simulink model "UnstablePlant"  (R2017b)
settings: Solver=VariableStepAuto  StartTime=0.0  StopTime=10.0  RelTol=1e-3
values from neighbouring files (symbols this model uses):
  Kp = 0.3    [open_loop.m]
  Ts = 0.005    [closed_loop.m]    (also in open_loop.m)
settings Model: Creator=tomas  LastModifiedBy=tomas

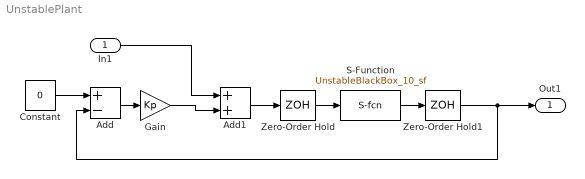
== system UnstablePlant ==
  In1 : Inport
  Add : Sum  Inputs=+-
  Add1 : Sum
  Constant : Constant  Value=0
  Gain : Gain  Gain=Kp
  S-Function : S-Function  FunctionName=UnstableBlackBox_10_sf  SFunctionDeploymentMode=off  EnableBusSupport=off  SFcnStateName=DWORK0
      settings: SFcnIsStateOwnerBlock=on
  Zero-Order Hold : ZeroOrderHold  SampleTime=Ts
  Zero-Order Hold1 : ZeroOrderHold  SampleTime=Ts
  Out1 : Outport
  wires:
  S-Function/1 -> Zero-Order Hold1/1
  Zero-Order Hold/1 -> S-Function/1
  In1/1 -> Add1/1
  Zero-Order Hold1/1 -> Add/2, Out1/1
  Constant/1 -> Add/1
  Add1/1 -> Zero-Order Hold/1
  Add/1 -> Gain/1
  Gain/1 -> Add1/2
